simulink library "lib_drive_cycle"  (Simulink 7.9)
settings: Solver=ode45  SolverMode=SingleTasking  StartTime=0.0  StopTime=10.0  RelTol=1e-3
undefined symbols (not defined in the file or in its folder): cyc_avg_time, cyc_cargo_mass, cyc_elevation_init, cyc_filter_bool, cyc_grade, cyc_mph
libraries: lib_drive_cycle x1
settings Model: Creator=mokeefe  LastModifiedBy=mokeefe  ModifiedComment=mokeefe -- Fri Mar 23 09:55:10 2012 -- Version 1.21
settings Model: ModifiedHistory=|
  | mokeefe -- Fri Mar 23 09:55:10 2012 -- Version 1.21
  | 
  | 
  | mokeefe -- Fri Mar 23 09:54:37 2012 -- Version 1.20
  | Upgraded mask variable reference from @1 to name of mask variable (super-smooth, no lag-trace)
  | 
  | mokeefe -- Fri Mar 23 09:52:49 2012 -- Version 1.19
  | updated repeated cycle vehicle cargo mass vs. distance, repeated cycle vehicle speed vs time, repeated grade vs distance. Changed mask initialization @1 to variable name.
  | 
  | kharalds -- Wed Aug 06 11:07:07 2003 -- Version 1.18
  | removed cyc_elevation_init from ambient presure calc
  | 
  | 
  | kharalds -- Wed Aug 06 10:53:50 2003 -- Version 1.17
  | revised height scale factor in ambient pressure calc
  | 
  | 
  | tmarkel -- Wed Jul 30 14:19:45 2003 -- Version 1.16
  | fixed bad link for ambient pressure calc
  | 
  | 
  | tmarkel -- Wed Jun 04 13:53:01 2003 -- Version 1.15
  | 
  | added calc and to workspace for ambient pressure as a function of elevation
  | 
  | 
  | mokeefe -- Thu Apr 18 08:26:19 2002 -- Version 1.14
  | saving the model:
  | o "without the model browser open"
  | o with only top-level screen visible
  | o with "fit to view" enabled
  | o with "status bar" off and "toolbar" off
  | o with "prompt to update model history with each save" on
  | 
  | mokeefe -- Thu Apr 18 08:26:08 2002 -- Version 1.13
  | saving the model:
  | o "without the model browser open"
  | o with only top-level screen visible
  | o with "fit to view" enabled
  | o with "status bar" off and "toolbar" off
  | o with "prompt to update model history with each save" on

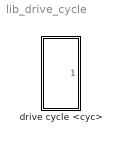
== system lib_drive_cycle ==
  drive cycle <cyc> : Subsystem
      mask Display: image(imread('bdi_cyc.jpg'))

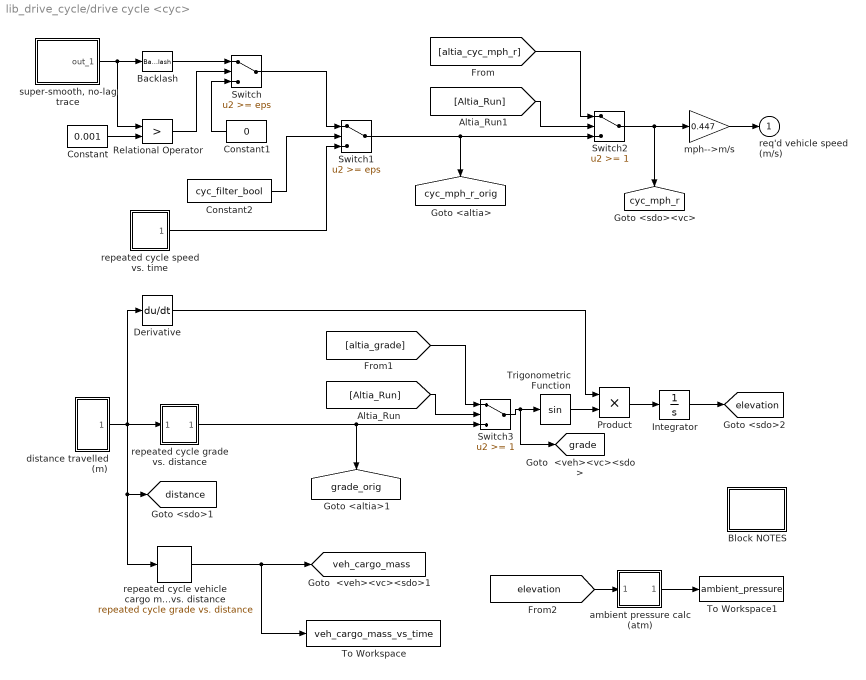
== system lib_drive_cycle/drive cycle <cyc> ==
  Backlash : Backlash  BacklashWidth=0.5
  Block NOTES : Subsystem
      mask Display: disp('Block\nNOTES')
  Constant : Constant  Value=0.001
  Constant1 : Constant  Value=0
  Constant2 : Constant  Value=cyc_filter_bool
  Derivative : Derivative
  Integrator : Integrator  InitialCondition=cyc_elevation_init
  Product : Product  SaturateOnIntegerOverflow=on  RndMeth=Zero  InputSameDT=on  OutDataTypeStr=Inherit: Same as first input
  Relational Operator : RelationalOperator  Operator=>  InputSameDT=on
  Switch : Switch  Threshold=eps  SaturateOnIntegerOverflow=on  InputSameDT=on
  Switch1 : Switch  Threshold=eps  SaturateOnIntegerOverflow=on  InputSameDT=on
  Switch2 : Switch  Threshold=1  SaturateOnIntegerOverflow=on  InputSameDT=on
  Switch3 : Switch  Threshold=1  SaturateOnIntegerOverflow=on  InputSameDT=on
  To Workspace : ToWorkspace  VariableName=veh_cargo_mass_vs_time  SampleTime=-1
  To Workspace1 : ToWorkspace  VariableName=ambient_pressure  SampleTime=-1
  Trigonometric Function : Trigonometry
  ambient pressure calc (atm) : Subsystem
  distance travelled (m) : Subsystem
  mph-->m/s : Gain  Gain=0.447  SaturateOnIntegerOverflow=on  OutDataTypeStr=Inherit: Same as input  ParamDataTypeStr=Inherit: Same as input
  repeated cycle grade vs. distance : Subsystem  mask(Repeating table){t=cyc_grade(:,1), y=cyc_grade(:,2)}
      mask prompts: t "Input values:"; y "Output values:"
      mask help:
      | Repeating table.
      | Enter values of input and output for first cycle.
      mask init:
      | period = max(t);
      mask Help: Repeats cycle given in table. Input values should be monotonically increasing.
  repeated cycle speed vs. time : Subsystem  mask(Repeating table){t=cyc_mph(:,1), y=cyc_mph(:,2)}
      mask prompts: t "Time values:"; y "Output values:"
      mask help:
      | Repeating table.
      | Enter values of time and output for first cycle.
      mask init:
      | period = max(t);
      mask Help: Repeats cycle given in table. Time values should be monotonically increasing.
  repeated cycle vehicle cargo mass vs. distance : lib_drive_cycle/drive cycle <cyc>/repeated cycle grade vs. distance  t=cyc_cargo_mass(:,1)  y=cyc_cargo_mass(:,2)
  "super-smooth, no-lag trace" : Subsystem  mask(Smooth Cycle){t=cyc_mph(:,1), y=cyc_mph(:,2), avgtime=cyc_avg_time}
      mask prompts: t "Time vector for trace (s):"; y "Speed vector for trace (km/hr):"; avgtime "Averaging time (s):"
      mask help: Smooth Cycle
      mask init:
      | period = max(t);,
      mask Display: disp('SMOOTH\nCYCLE')
  req'd vehicle speed (m/s) : Outport  InitialOutput=0
  tag scope: cyc_mph_r=global, cyc_mph_r_orig=global, distance=global, elevation=global, grade=global, grade_orig=global, veh_cargo_mass=global
  wires:
  repeated cycle grade vs. distance/1(out_1) -> [grade_orig], Switch3/3
  distance travelled (m)/1(Out1) -> repeated cycle grade vs. distance/1(distance travelled (m)), Derivative/1, [distance], repeated cycle vehicle cargo mass vs. distance/1
  Switch3/1 -> Trigonometric Function/1, [grade]
  Integrator/1 -> [elevation]
  Trigonometric Function/1 -> Product/2
  Derivative/1 -> Product/1
  Product/1 -> Integrator/1
  Switch1/1 -> Switch2/3, [cyc_mph_r_orig]
  repeated cycle speed vs. time/1(out_1) -> Switch1/3
  Switch/1 -> Switch1/1
  "super-smooth, no-lag trace"/1(out_1) -> Backlash/1, Relational Operator/1
  Constant/1 -> Relational Operator/2
  Backlash/1 -> Switch/1
  Relational Operator/1 -> Switch/2
  Constant1/1 -> Switch/3
  Constant2/1 -> Switch1/2
  Switch2/1 -> [cyc_mph_r], mph-->m/s/1
  mph-->m/s/1 -> req'd vehicle speed (m/s)/1
  [altia_cyc_mph_r] -> Switch2/1
  [Altia_Run] -> Switch2/2
  [altia_grade] -> Switch3/1
  [Altia_Run] -> Switch3/2
  repeated cycle vehicle cargo mass vs. distance/1 -> [veh_cargo_mass], To Workspace/1
  ambient pressure calc (atm)/1(Out1) -> To Workspace1/1
  [elevation] -> ambient pressure calc (atm)/1(elevation)

== system lib_drive_cycle/drive cycle <cyc>/Block NOTES ==
  note: This block determines the speed required of the vehicle.  If cyc_filter_bool
      | is true, a centered-in-time average of the trace, with backlash, is required of
      | the vehicle.  This may be useful to smooth out jumps in the trace.  Otherwise,
      | the trace, exactly as published, is required of the vehicle.
      | This block also determines the roadway grade of the cycle and the
      | elevation as a function of the distance travelelled

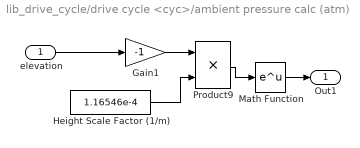
== system lib_drive_cycle/drive cycle <cyc>/ambient pressure calc (atm) ==
  elevation : Inport
  Gain1 : Gain  Gain=-1  SaturateOnIntegerOverflow=on  OutDataTypeStr=Inherit: Same as input  ParamDataTypeStr=Inherit: Same as input
  Height Scale Factor (1/m) : Constant  Value=1.16546e-4
  Math Function : Math  SaturateOnIntegerOverflow=on
  Product9 : Product  SaturateOnIntegerOverflow=on  RndMeth=Zero  InputSameDT=on  OutDataTypeStr=Inherit: Same as first input
  Out1 : Outport
  wires:
  Product9/1 -> Math Function/1
  elevation/1 -> Gain1/1
  Gain1/1 -> Product9/1
  Height Scale Factor (1/m)/1 -> Product9/2
  Math Function/1 -> Out1/1

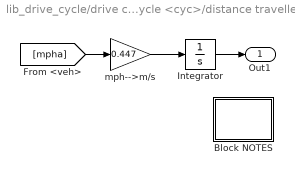
== system lib_drive_cycle/drive cycle <cyc>/distance travelled (m) ==
  Block NOTES : Subsystem
      mask Display: disp('Block\nNOTES')
  Integrator : Integrator
  mph-->m/s : Gain  Gain=0.447  SaturateOnIntegerOverflow=on  OutDataTypeStr=Inherit: Same as input  ParamDataTypeStr=Inherit: Same as input
  Out1 : Outport  InitialOutput=0
  wires:
  Integrator/1 -> Out1/1
  [mpha] -> mph-->m/s/1
  mph-->m/s/1 -> Integrator/1

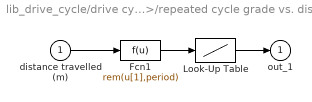
== system lib_drive_cycle/drive cycle <cyc>/repeated cycle grade vs. distance ==
  distance travelled (m) : Inport
  Fcn1 : Fcn  Expr=rem(u[1],period)
  Look-Up Table : Lookup  InputValues=t  Table=y  SaturateOnIntegerOverflow=on
  out_1 : Outport  InitialOutput=0
  wires:
  distance travelled (m)/1 -> Fcn1/1
  Fcn1/1 -> Look-Up Table/1
  Look-Up Table/1 -> out_1/1

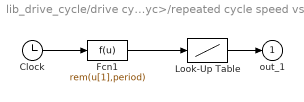
== system lib_drive_cycle/drive cycle <cyc>/repeated cycle speed vs. time ==
  Clock : Clock
  Fcn1 : Fcn  Expr=rem(u[1],period)
  Look-Up Table : Lookup  InputValues=t  Table=y  SaturateOnIntegerOverflow=on
  out_1 : Outport  InitialOutput=0
  wires:
  Fcn1/1 -> Look-Up Table/1
  Clock/1 -> Fcn1/1
  Look-Up Table/1 -> out_1/1

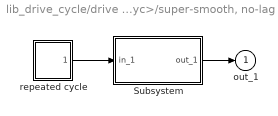
== system lib_drive_cycle/drive cycle <cyc>/super-smooth, no-lag trace ==
  Subsystem : Subsystem  mask(Running Average){n=avgtime}
      mask prompts: n "Averaging Time (s)"
      mask help: Running Average
      mask Help: Output is the average of the last (Averaging Time) seconds of input.
      mask Display: disp('Running\nAverage')
  repeated cycle : Subsystem
  out_1 : Outport  InitialOutput=0
  wires:
  Subsystem/1(out_1) -> out_1/1
  repeated cycle/1(out_1) -> Subsystem/1(in_1)

== system lib_drive_cycle/drive cycle <cyc>/distance travelled (m)/Block NOTES ==
  note: This block calculates the distance travelled by the
      |  vehicle based on the achieved speed.

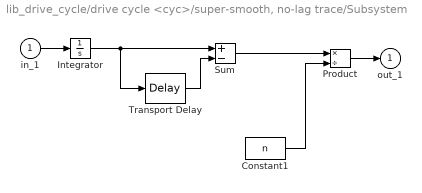
== system lib_drive_cycle/drive cycle <cyc>/super-smooth, no-lag trace/Subsystem ==
  in_1 : Inport
  Constant1 : Constant  Value=n
  Integrator : Integrator
  Product : Product  Inputs=*/  SaturateOnIntegerOverflow=on  RndMeth=Zero  InputSameDT=on  OutDataTypeStr=Inherit: Same as first input
  Sum : Sum  Inputs=+-  SaturateOnIntegerOverflow=on  InputSameDT=on  OutDataTypeStr=Inherit: Same as first input
  Transport Delay : TransportDelay  DelayTime=n
  out_1 : Outport  InitialOutput=0
  wires:
  Constant1/1 -> Product/2
  Product/1 -> out_1/1
  in_1/1 -> Integrator/1
  Sum/1 -> Product/1
  Transport Delay/1 -> Sum/2
  Integrator/1 -> Transport Delay/1, Sum/1

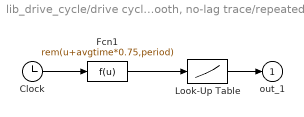
== system lib_drive_cycle/drive cycle <cyc>/super-smooth, no-lag trace/repeated cycle ==
  Clock : Clock
  Fcn1 : Fcn  Expr=rem(u+avgtime*0.75,period)
  Look-Up Table : Lookup  InputValues=t  Table=y  SaturateOnIntegerOverflow=on
  out_1 : Outport  InitialOutput=0
  wires:
  Look-Up Table/1 -> out_1/1
  Clock/1 -> Fcn1/1
  Fcn1/1 -> Look-Up Table/1
